simulink model "dualbridge"  (R2025b)
settings: Solver=VariableStepAuto  StartTime=0.0  StopTime=0.1  RelTol=1e-3
libraries: spsSeriesRLCBranchLib x6, spsIGBTDiodeLib x4, spsMosfetLib x4, spsDCVoltageSourceLib x2, spsPWMGeneratorDCDCLib x2, spsCurrentMeasurementLib x1, spsMeanLib x1, spsVariableRatioTransformerLib x1, spsVoltageMeasurementLib x1, spspowerguiLib x1
settings Model: Creator=hp  LastModifiedBy=admin

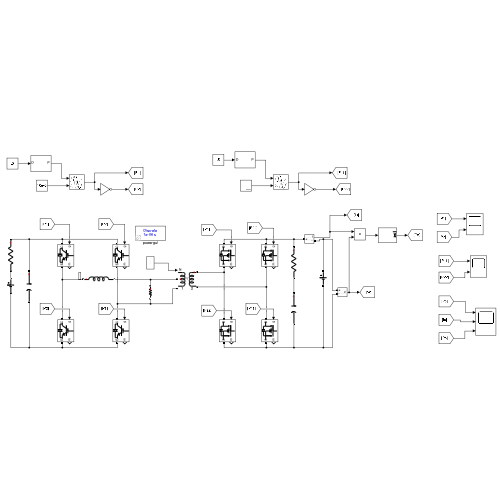
[thumbnail: Simulink's stored preview of the top-level diagram]
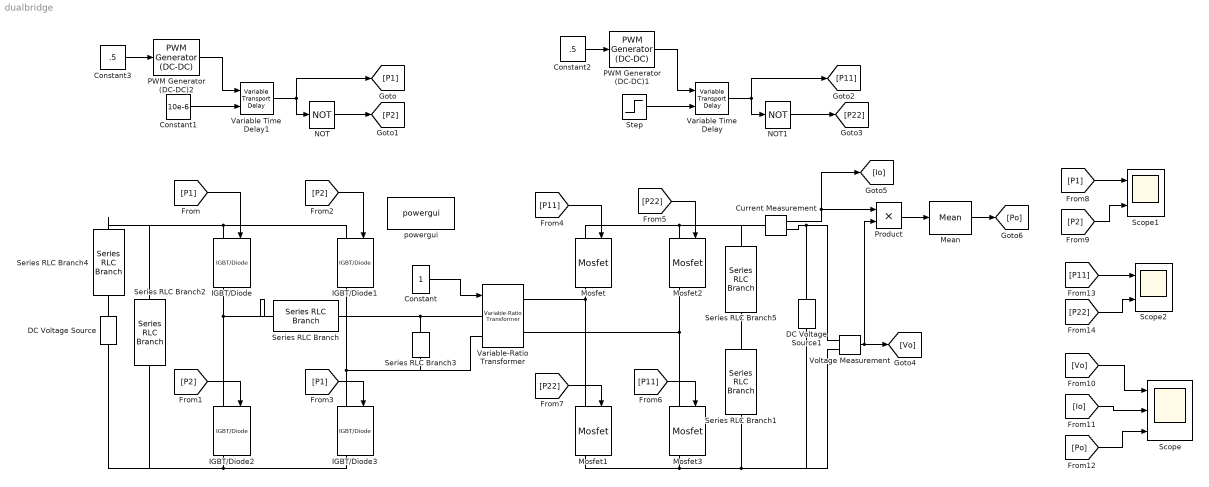
== system dualbridge ==
  Constant : Constant
  Constant1 : Constant  Value=10e-6
  Constant2 : Constant  Value=.5
  Constant3 : Constant  Value=.5
  Current Measurement : spsCurrentMeasurementLib/Current Measurement  PhasorSimulation=off  OutputType=Complex  PSBequivalent=0
  DC Voltage Source : spsDCVoltageSourceLib/DC Voltage Source  Amplitude=50  Measurements=None
  DC Voltage Source1 : spsDCVoltageSourceLib/DC Voltage Source  Amplitude=48  Measurements=None
  IGBT/Diode{,1..3} (4 alike) : spsIGBTDiodeLib/IGBT//Diode  Ron=1e-3  Rs=1e5  Cs=inf  Measurements=on
  Mean : spsMeanLib/Mean  Freq=50  Vinit=0  Ts=0
  Mosfet{,1..3} (4 alike) : spsMosfetLib/Mosfet  Ron=0.1  Lon=0  Rd=0.01  Vfd=0  IC=0  Rs=1e5  Cs=inf  Measurements=on
  NOT : Logic  Operator=NOT  IconShape=distinctive  AllPortsSameDT=off  OutDataTypeStr=boolean
  NOT1 : Logic  Operator=NOT  IconShape=distinctive  AllPortsSameDT=off  OutDataTypeStr=boolean
  PWM Generator (DC-DC)1 : spsPWMGeneratorDCDCLib/PWM Generator (DC-DC)  Fsw=20000  Ts=1e-7
  PWM Generator (DC-DC)2 : spsPWMGeneratorDCDCLib/PWM Generator (DC-DC)  Fsw=20000  Ts=1e-7
  Product : Product
  Scope : Scope  NumInputPorts=3
      settings: Title=Output Voltage  ActiveDisplayYMinimum=45  ActiveDisplayYMaximum=50
  Scope1 : Scope  NumInputPorts=2
      settings: ActiveDisplayYMinimum=-0.12499999999999997  ActiveDisplayYMaximum=1.125
  Scope2 : Scope  NumInputPorts=2
      settings: ActiveDisplayYMinimum=-0.12499999999999997  ActiveDisplayYMaximum=1.125  DataLoggingVariableName=ScopeData2
  Series RLC Branch : spsSeriesRLCBranchLib/Series RLC Branch  LConnTagsString=__new0  RConnTagsString=__new0  BranchType=L  Resistance=0.01  Inductance=100e-6  SetiL0=off  InitialCurrent=0  Capacitance=1e-6  Setx0=off  InitialVoltage=0  Measurements=None
  Series RLC Branch1 : spsSeriesRLCBranchLib/Series RLC Branch  LConnTagsString=__new0  RConnTagsString=__new0  BranchType=C  Resistance=1  Inductance=1e-3  SetiL0=off  InitialCurrent=0  Capacitance=1000e-6  Setx0=off  InitialVoltage=0  Measurements=None
  Series RLC Branch2 : spsSeriesRLCBranchLib/Series RLC Branch  LConnTagsString=__new0  RConnTagsString=__new0  BranchType=C  Resistance=1  Inductance=1e-3  SetiL0=off  InitialCurrent=0  Capacitance=1000e-6  Setx0=off  InitialVoltage=0  Measurements=None
  Series RLC Branch3 : spsSeriesRLCBranchLib/Series RLC Branch  LConnTagsString=__new0  RConnTagsString=__new0  BranchType=R  Resistance=100  Inductance=100e-6  SetiL0=off  InitialCurrent=0  Capacitance=1e-6  Setx0=off  InitialVoltage=0  Measurements=None
  Series RLC Branch4 : spsSeriesRLCBranchLib/Series RLC Branch  LConnTagsString=__new0  RConnTagsString=__new0  BranchType=R  Resistance=1e-3  Inductance=1e-3  SetiL0=off  InitialCurrent=0  Capacitance=1000e-6  Setx0=off  InitialVoltage=0  Measurements=None
  Series RLC Branch5 : spsSeriesRLCBranchLib/Series RLC Branch  LConnTagsString=__new0  RConnTagsString=__new0  BranchType=R  Resistance=1e-3  Inductance=1e-3  SetiL0=off  InitialCurrent=0  Capacitance=1000e-6  Setx0=off  InitialVoltage=0  Measurements=None
  Step : Step  Time=0.05  Before=15e-6  After=5e-6  SampleTime=0
  Variable Time Delay : VariableTransportDelay  MaximumDelay=10
  Variable Time Delay1 : VariableTransportDelay  MaximumDelay=10
  Variable-Ratio Transformer : spsVariableRatioTransformerLib/Variable-Ratio Transformer
      settings: LibrarySourceBlock=|
      | sps_lib/Passives/Variable-Ratio
      | Transformer
  Voltage Measurement : spsVoltageMeasurementLib/Voltage Measurement  PhasorSimulation=off  OutputType=Complex  PSBequivalent=0
  powergui : spspowerguiLib/powergui  Priority=1  SimulationMode=Discrete  SampleTime=1e-6  frequency=60  Iterations=50  frequencyindice=0  Pbase=100e6  ErrMax=1e-4  UnitsV=kV  UnitsW=MW  buscounter=0  FunctionMessages=off  echomessages=off  EnableUseOfTLC=off  CurrentSourceSwitches=off  DisableSnubberDevices=off  DisableRonSwitches=off  DisableVfSwitches=off  DisplayEquations=off  AutomaticDiscreteSolvers=off  SolverType=Tustin/Backward Euler (TBE)  Interpol=off  ExternalGateDelay=off  methode=off  Ts=100  x0status=blocks  SPID=on  SwTol=0  HookPort=off  NonlinearTolerance=1e-4  nMaxIteration=100  ContinueOnMaxIteration=off  RestoreLinks=warning  ResistiveCurrentMeasurement=off  Frange=[0:2:500]  Ylog=off  Xlog=on  ShowGrid=off  save=off  variable=ZData  structure=0  ZoomFFT=off  StartTime=0.0  cycles=1  DisplayStyle=1  fundamental=60  FreqAxis=off  MaxFrequency=1000  frequencyindicesteady=1  RmsSteady=1  display=off
  wires:
  NOT/1 -> [P2]
  [P1] -> IGBT/Diode3/1
  [P2] -> IGBT/Diode1/1
  [P1] -> IGBT/Diode/1
  [P2] -> IGBT/Diode2/1
  Voltage Measurement/1 -> Product/2, [Vo]
  Constant/1 -> Variable-Ratio Transformer/1
  Current Measurement/1 -> [Io], Product/1
  Product/1 -> Mean/1
  Mean/1 -> [Po]
  NOT1/1 -> [P22]
  [P22] -> Mosfet1/1
  [P11] -> Mosfet3/1
  [P22] -> Mosfet2/1
  [P11] -> Mosfet/1
  [P1] -> Scope1/1
  [P2] -> Scope1/2
  [Io] -> Scope/2
  [Vo] -> Scope/1
  [Po] -> Scope/3
  [P11] -> Scope2/1
  [P22] -> Scope2/2
  Variable Time Delay/1 -> [P11], NOT1/1
  Step/1 -> Variable Time Delay/2
  PWM Generator (DC-DC)1/1 -> Variable Time Delay/1
  Constant2/1 -> PWM Generator (DC-DC)1/1
  PWM Generator (DC-DC)2/1 -> Variable Time Delay1/1
  Constant3/1 -> PWM Generator (DC-DC)2/1
  Constant1/1 -> Variable Time Delay1/2
  Variable Time Delay1/1 -> [P1], NOT/1
  connections:
  IGBT/Diode2/LConn1 -- Series RLC Branch/LConn1 -- IGBT/Diode/RConn1
  IGBT/Diode3/LConn1 -- Variable-Ratio Transformer/LConn2 -- Series RLC Branch3/RConn1 -- IGBT/Diode1/RConn1
  IGBT/Diode/LConn1 -- Series RLC Branch4/LConn1 -- Series RLC Branch2/LConn1 -- IGBT/Diode1/LConn1
  IGBT/Diode2/RConn1 -- Series RLC Branch2/RConn1 -- DC Voltage Source/LConn1 -- IGBT/Diode3/RConn1
  Series RLC Branch/RConn1 -- Series RLC Branch3/LConn1 -- Variable-Ratio Transformer/LConn1
  Mosfet1/LConn1 -- Variable-Ratio Transformer/RConn1 -- Mosfet/RConn1
  Mosfet3/LConn1 -- Variable-Ratio Transformer/RConn2 -- Mosfet2/RConn1
  Mosfet/LConn1 -- Series RLC Branch5/LConn1 -- Current Measurement/LConn1 -- Mosfet2/LConn1
  Mosfet1/RConn1 -- DC Voltage Source1/LConn1 -- Voltage Measurement/LConn2 -- Series RLC Branch1/RConn1 -- Mosfet3/RConn1
  Current Measurement/RConn1 -- DC Voltage Source1/RConn1 -- Voltage Measurement/LConn1
  Series RLC Branch4/RConn1 -- DC Voltage Source/RConn1
  Series RLC Branch5/RConn1 -- Series RLC Branch1/LConn1
